simulink model "MtrCtrl_24V_2018"  (R2018b)
settings: Solver=FixedStepDiscrete  StartTime=0.0  StopTime=1  FixedStep=1e-6  RelTol=1e-3
values from neighbouring files (symbols this model uses):
  B = 0.001889    [MtrCtrl_v01.sldd]
  C_LUT_AngleTable_sng_Null = 0.0015339807878856412 0.0030679615757712823 0.0046019423636569235 0.0061359231515425647 0.0076699039394282058 0.009203884727313847 0.010737865515199488 0.012271846303085129 0.013805827090970771 0.015339807878856412 0.016873788666742051 0.018407769454627694 0.019941750242513337 0.021475731030398976 0.023009711818284616 0.024543692606170259 0.0260776733940559 0.027611654181941541 0.02914563496982718    [MtrCtrl_v01.sldd]
  C_LUT_SinTable_sng_Null = 0.0015339801862847655 0.0030679567629659761 0.0046019261204485705 0.0061358846491544753 0.007669828739531097 0.00920375478205982 0.010737659167264491 0.012271538285719925 0.013805388528060391 0.0153392062849881 0.01687298794728171 0.01840672990580482 0.019940428551514441 0.021474080275469508 0.023007681468839369 0.024541228522912288 0.0260747178291039 0.02760814577896574 0.029141508764193722 0.030    [MtrCtrl_v01.sldd]
  C_MATH_OneOverSqrtThree_s32n31_Null = 0.57735026918962584    [MtrCtrl_v01.sldd]
  C_MATH_Pi_u32n30_Null = 3.1415926535897931    [MtrCtrl_v01.sldd]
  C_MATH_SqrtThreeOverThree_s32n31_Null = 0.57735026918962573    [MtrCtrl_v01.sldd]
  C_PMSM_CurQKi_u32n31_null = 0.15707963267949    [MtrCtrl_v01.sldd]
  C_PMSM_CurQKp_u32n31_null = 19.949113350295185    [MtrCtrl_v01.sldd]
  C_PMSM_Flux_u32n32_Vs = 0.192    [MtrCtrl_v01.sldd]
  C_PMSM_Ls_pu = 0.398982267005904    [MtrCtrl_v01.sldd]
  C_PMSM_PolePairs_u8_Null = 4.0    [MtrCtrl_v01.sldd]
  Flux = 0.192    [MtrCtrl_v01.sldd]
  IBase_A = 2000.0    [MtrCtrl_v01.sldd]
  J = 0.011    [MtrCtrl_v01.sldd]
  K_CCM_MRASEna_bool_Flg = 0.0    [MtrCtrl_v01.sldd]
  K_SVM_DefultDuty_s32n31_Null = 0.25    [MtrCtrl_v01.sldd]
  KCCM_VirPosn_flg = 0.0    [MtrCtrl_v01.sldd]
  KCCM_VoltModeEna_Flg = 0.0    [MtrCtrl_v01.sldd]
  Kis = 114583.3333333333    [MtrCtrl_v01.sldd]
  KSMO_EnaEst_Flg = 0.0    [MtrCtrl_v01.sldd]
  Kt = 1.1520000000000001    [MtrCtrl_v01.sldd]
  Ld = 0.000635    [MtrCtrl_v01.sldd]
  LPF_coefg = 0.01    [MtrCtrl_v01.sldd]
  Lq = 0.000685    [MtrCtrl_v01.sldd]
  Ls = 0.000635    [MtrCtrl_v01.sldd]
  OneOverUBase_V = 0.0016666666666666668    [MtrCtrl_v01.sldd]
  Pp = 4.0    [MtrCtrl_v01.sldd]
  Rs = 0.05    [MtrCtrl_v01.sldd]
  SecPerRnd = 0.6    [MtrCtrl_v01.sldd]
  SMOGain_V = 323.31615074619043    [MtrCtrl_v01.sldd]
  Ts = 1.0E-6    [MtrCtrl_v01.sldd]
  TsCtrl = 1.0E-6    [MtrCtrl_v01.sldd]
  UBase_V = 600.0    [MtrCtrl_v01.sldd]
  wmBase_rps = 314.15926535897933    [MtrCtrl_v01.sldd]
undefined symbols (not defined in the file or in its folder): DiscIntNeverNeededParam, Ion, Lithium, sinTable
libraries: powerlib x39, simulink x17, ee_lib x16, nesl_utility x6, simulink_extras x2, eePmsmFwController x1, electricdrivelib x1, fl_lib x1
(part 4 of 5)

== system MtrCtrl_24V_2018/CurLpCtrl/Subsystem10/Subsystem ==
  idqRef : Inport  OutDataTypeStr=fixdt(1,32,31)
  vdq : Inport  Port=2  OutDataTypeStr=fixdt(1,32,31)
  VphMax : Inport  Port=3  OutDataTypeStr=fixdt(0,32,32)
  Cartesian to Polar : Subsystem  Tag=DecoupledSystem
  Constant : Constant  Value=C_MATH_Pi_u32n30_Null  OutDataTypeStr=fixdt(0,32,30)  SampleTime=-1
  Demux : Demux  Outputs=2
  Discrete-Time Integrator : DiscreteIntegrator  IntegratorMethod=Integration: Backward Euler  gainval=5  InitialCondition=1  SampleTime=-1  OutDataTypeStr=fixdt(1,32,28)  ICPrevOutput=DiscIntNeverNeededParam  ICPrevScaledInput=DiscIntNeverNeededParam
  Gain : Gain  Gain=50  OutDataTypeStr=fixdt(1,32,25)
  Gain1 : Gain  Gain=10  OutDataTypeStr=fixdt(1,32,25)
  Gain2 : Gain  Gain=2
  Modulation index threshold : Constant  Value=C_MATH_SqrtThreeOverThree_s32n31_Null  OutDataTypeStr=fixdt(0,32,31)  SampleTime=-1
  Modulation index threshold1 : Constant  Value=3.24  OutDataTypeStr=fixdt(0,32,30)  SampleTime=-1
  Mux : Mux  Inputs=2
  Polar to Cartesian : Subsystem  Tag=DecoupledSystem
  Product : Product  OutDataTypeStr=fixdt(1,32,28)
  Saturation : Saturate  UpperLimit=1  LowerLimit=0  OutDataTypeStr=fixdt(1,32,28)
  Subsystem1 : Subsystem
  Sum : Sum  Inputs=|-+  OutDataTypeStr=fixdt(1,32,30)
  Sum1 : Sum  Inputs=|-+  OutDataTypeStr=fixdt(1,32,28)
  Sum2 : Sum  Inputs=|-+  OutDataTypeStr=fixdt(1,32,28)
  Sum3 : Sum  Inputs=-+  OutDataTypeStr=fixdt(1,32,28)
  Sum4 : Sum  Inputs=|++  OutDataTypeStr=fixdt(1,32,25)
  Unit Delay : UnitDelay  SampleTime=-1  HasFrameUpgradeWarning=on
  idqRefFW : Outport  VectorParamsAs1DForOutWhenUnconnected=off
  wires:
  Product/1 -> Sum2/1
  Sum1/1 -> Product/1
  Gain1/1 -> Sum4/2
  Cartesian to Polar/1(Out1) -> Polar to Cartesian/1(In1)
  Subsystem1/1(M) -> Sum/1
  Sum/1 -> Gain/1
  Discrete-Time Integrator/1 -> Saturation/1, Sum3/1
  Unit Delay/1 -> Gain1/1
  Cartesian to Polar/2(Out2) -> Sum1/1
  Polar to Cartesian/2(Out2) -> Mux/2
  Mux/1 -> idqRefFW/1
  Gain/1 -> Sum4/1
  VphMax/1 -> Subsystem1/2(VphMax)
  Modulation index threshold/1 -> Gain2/1
  Saturation/1 -> Product/2, Sum3/2
  Demux/2 -> Cartesian to Polar/2(In2)
  Demux/1 -> Cartesian to Polar/1(In1)
  idqRef/1 -> Demux/1
  Polar to Cartesian/1(Out1) -> Mux/1
  Constant/1 -> Sum1/2, Sum2/2
  Sum3/1 -> Unit Delay/1
  vdq/1 -> Subsystem1/1(vdq)
  Sum2/1 -> Polar to Cartesian/2(In2)
  Sum4/1 -> Discrete-Time Integrator/1
  Gain2/1 -> Sum/2

== system MtrCtrl_24V_2018/CurLpCtrl/Subsystem2/Subsystem1 ==
  In1 : Inport  OutDataTypeStr=fixdt(0,32,0)
  Constant7 : Constant  Value=2*pi  OutDataTypeStr=fixdt(0,32,0)
  Mod : Math  Operator=mod  SaturateOnIntegerOverflow=on
  Out1 : Outport
  wires:
  Mod/1 -> Out1/1
  In1/1 -> Mod/1
  Constant7/1 -> Mod/2

== system MtrCtrl_24V_2018/CurLpCtrl/Subsystem2/Subsystem2 ==
  FilterIn : Inport  OutDataTypeStr=fixdt(1,32,31)
  Rest : Inport  Port=2  OutDataTypeStr=fixdt(1,32,0)
  Add : Sum  Inputs=+-  OutDataTypeStr=fixdt(1,32,31)
  Add1 : Sum  OutDataTypeStr=fixdt(1,32,31)
  Constant : Constant  Value=LPF_coefg  OutDataTypeStr=fixdt(0,32,31)
  Delay : Delay  DelayLength=1  ExternalReset=Either
      settings: InputPortMap=u0,r5
  Product : Product  OutDataTypeStr=fixdt(1,32,31)
  FilterOut : Outport
  wires:
  FilterIn/1 -> Add/1
  Add/1 -> Product/2
  Product/1 -> Add1/1
  Add1/1 -> Delay/1, FilterOut/1
  Delay/1 -> Add/2, Add1/2
  Rest/1 -> Delay/2
  Constant/1 -> Product/1

== system MtrCtrl_24V_2018/CurLpCtrl/Subsystem2/Subsystem3 ==
  ParkPosn : Inport  OutDataTypeStr=fixdt(1,32,28)
  1-D Lookup Table : Lookup_n-D  NumberOfTableDimensions=1  BreakpointsForDimension1=sinTable(2,:)  BeginIndexSearchUsingPreviousIndexResult=on  Table=sinTable(1,:)  ExtrapMethod=Clip  UseLastTableValue=on  InternalRulePriority=Speed  OutDataTypeStr=fixdt(0,32,31)  RndMeth=Simplest  InputSameDT=on
  1-D Lookup Table1 : Lookup_n-D  NumberOfTableDimensions=1  BreakpointsForDimension1=sinTable(2,:)  BeginIndexSearchUsingPreviousIndexResult=on  Table=sinTable(1,:)  ExtrapMethod=Clip  UseLastTableValue=on  InternalRulePriority=Speed  OutDataTypeStr=fixdt(0,32,31)  RndMeth=Simplest  InputSameDT=on
  Add : Sum  OutDataTypeStr=fixdt(1,32,26)
  Chart : Stateflow chart  TreatAsAtomicUnit=on
  Constant1 : Constant  Value=0  OutDataTypeStr=fixdt(1,32,4)
  Gain : Gain  Gain=4  OutDataTypeStr=fixdt(1,32,26)
  Product : Product  OutDataTypeStr=fixdt(1,32,30)  RndMeth=Simplest
  Product1 : Product  OutDataTypeStr=fixdt(1,32,30)
  Scope : Scope  NumInputPorts=3
  SinTheta : Outport
  CosTheta : Outport  Port=2
  wires:
  ParkPosn/1 -> Gain/1
  Gain/1 -> Add/2
  Constant1/1 -> Add/1
  Product/1 -> Scope/1, SinTheta/1
  Product1/1 -> Scope/2, CosTheta/1
  Add/1 -> Scope/3, Chart/1(Angle)
  Chart/1(SinAngle) -> 1-D Lookup Table/1
  Chart/3(CosAngle) -> 1-D Lookup Table1/1
  1-D Lookup Table/1 -> Product/1
  Chart/2(SinSign) -> Product/2
  1-D Lookup Table1/1 -> Product1/1
  Chart/4(CosSign) -> Product1/2

== system MtrCtrl_24V_2018/CurLpCtrl/Subsystem2/Subsystem4 ==
  FilterIn : Inport  OutDataTypeStr=fixdt(1,32,31)
  Rest : Inport  Port=2  OutDataTypeStr=fixdt(1,32,0)
  Add : Sum  Inputs=+-  OutDataTypeStr=fixdt(1,32,31)
  Add1 : Sum  OutDataTypeStr=fixdt(1,32,31)
  Constant : Constant  Value=LPF_coefg  OutDataTypeStr=fixdt(0,32,31)
  Delay : Delay  DelayLength=1  ExternalReset=Either
      settings: InputPortMap=u0,r5
  Product : Product  OutDataTypeStr=fixdt(1,32,31)
  FilterOut : Outport
  wires:
  Rest/1 -> Delay/2
  Delay/1 -> Add1/2, Add/2
  Add1/1 -> FilterOut/1, Delay/1
  Product/1 -> Add1/1
  Add/1 -> Product/2
  FilterIn/1 -> Add/1
  Constant/1 -> Product/1

== system MtrCtrl_24V_2018/CurLpCtrl/Subsystem2/Subsystem5 ==
  FilterIn : Inport  OutDataTypeStr=fixdt(1,32,22)
  Rest : Inport  Port=2  OutDataTypeStr=fixdt(1,32,0)
  Add : Sum  Inputs=+-  OutDataTypeStr=fixdt(1,32,23)
  Add1 : Sum  OutDataTypeStr=fixdt(1,32,22)
  Constant : Constant  Value=LPF_coefg  OutDataTypeStr=fixdt(0,32,38)
  Delay : Delay  DelayLength=1  ExternalReset=Either
      settings: InputPortMap=u0,r5
  Product : Product  OutDataTypeStr=fixdt(1,32,29)
  FilterOut : Outport
  wires:
  FilterIn/1 -> Add/1
  Add/1 -> Product/2
  Product/1 -> Add1/1
  Add1/1 -> Delay/1, FilterOut/1
  Delay/1 -> Add/2, Add1/2
  Rest/1 -> Delay/2
  Constant/1 -> Product/1

== system MtrCtrl_24V_2018/CurLpCtrl/Subsystem2/Z_alpha ==
  Salpha : Inport  OutDataTypeStr=int32
  Constant : Constant  OutDataTypeStr=fixdt(1,32,30)
  Constant1 : Constant  Value=-1  OutDataTypeStr=fixdt(1,32,30)
  Divide : Product  Inputs=*/  OutDataTypeStr=fixdt(1,32,30)
  E : Constant  Value=600  OutDataTypeStr=int32
  If : If  NumInputs=2  IfExpression=u1 > u2  ElseIfExpressions=u1 < -u2
  If Action Subsystem : Subsystem  TreatAsAtomicUnit=on
  If Action Subsystem1 : Subsystem  TreatAsAtomicUnit=on
  If Action Subsystem2 : Subsystem  TreatAsAtomicUnit=on
  Merge : Merge  Inputs=3
  ZalphaOut : Outport
  wires:
  Salpha/1 -> If/1, Divide/1
  E/1 -> If/2, Divide/2
  Divide/1 -> If Action Subsystem2/1(In1)
  If/1 -> If Action Subsystem/Action
  If Action Subsystem/1(ZalphaOut) -> Merge/1
  If/3 -> If Action Subsystem2/Action
  If/2 -> If Action Subsystem1/Action
  If Action Subsystem1/1(ZalphaOut) -> Merge/2
  If Action Subsystem2/1(ZalphaOut) -> Merge/3
  Merge/1 -> ZalphaOut/1
  Constant/1 -> If Action Subsystem/1(In1)
  Constant1/1 -> If Action Subsystem1/1(In1)

== system MtrCtrl_24V_2018/CurLpCtrl/Subsystem2/Z_alpha1 ==
  Salpha : Inport  OutDataTypeStr=int32
  Constant : Constant  OutDataTypeStr=fixdt(1,32,30)
  Constant1 : Constant  Value=-1  OutDataTypeStr=fixdt(1,32,30)
  Divide : Product  Inputs=*/  OutDataTypeStr=fixdt(1,32,30)
  E : Constant  Value=600  OutDataTypeStr=int32
  If : If  NumInputs=2  IfExpression=u1 > u2  ElseIfExpressions=u1 < -u2
  If Action Subsystem : Subsystem  TreatAsAtomicUnit=on
  If Action Subsystem1 : Subsystem  TreatAsAtomicUnit=on
  If Action Subsystem2 : Subsystem  TreatAsAtomicUnit=on
  Merge : Merge  Inputs=3
  ZalphaOut : Outport
  wires:
  Constant1/1 -> If Action Subsystem1/1(In1)
  Constant/1 -> If Action Subsystem/1(In1)
  Merge/1 -> ZalphaOut/1
  If Action Subsystem2/1(ZalphaOut) -> Merge/3
  If Action Subsystem1/1(ZalphaOut) -> Merge/2
  If/2 -> If Action Subsystem1/Action
  If/3 -> If Action Subsystem2/Action
  If Action Subsystem/1(ZalphaOut) -> Merge/1
  If/1 -> If Action Subsystem/Action
  Divide/1 -> If Action Subsystem2/1(In1)
  E/1 -> Divide/2, If/2
  Salpha/1 -> Divide/1, If/1

== system MtrCtrl_24V_2018/CurLpCtrl/Subsystem4/SinCos ==
  In1 : Inport  LockScale=on
  DTC_input_1 : DataTypeConversion  OutDataTypeStr=fixdt('double')  RndMeth=Nearest  LockScale=on
  DTC_output_1 : DataTypeConversion  OutDataTypeStr=fixdt(1,32,4)
  DTC_output_2 : DataTypeConversion  OutDataTypeStr=fixdt(0,32,31)
  ReplicaOfSource : Trigonometry  Operator=sincos
  Out1 : Outport  LockScale=on
  Out2 : Outport  Port=2  LockScale=on
  wires:
  In1/1 -> DTC_input_1/1
  DTC_output_1/1 -> Out1/1
  ReplicaOfSource/1 -> DTC_output_1/1
  ReplicaOfSource/2 -> DTC_output_2/1
  DTC_input_1/1 -> ReplicaOfSource/1
  DTC_output_2/1 -> Out2/1

== system MtrCtrl_24V_2018/CurLpCtrl/Subsystem8/F12 ==
  we : Inport
  Dlt_Ud_k : Inport  Port=2
  Dlt_Uq_k : Inport  Port=3
  Add{2..5} (4 alike) : Sum
  Constant1 : Constant  Value=-TsCtrl*Rs/Ls
  Constant14 : Constant  Value=-TsCtrl*Rs/Ls
  Constant16 : Constant  Value=TsCtrl/Ls
  Constant2 : Constant  Value=TsCtrl/Ls
  Discrete-Time Integrator : DiscreteIntegrator  SampleTime=-1  ICPrevOutput=DiscIntNeverNeededParam  ICPrevScaledInput=DiscIntNeverNeededParam
  Discrete-Time Integrator1 : DiscreteIntegrator  SampleTime=-1  ICPrevOutput=DiscIntNeverNeededParam  ICPrevScaledInput=DiscIntNeverNeededParam
  Gain6 : Gain  Gain=TsCtrl
  Gain7 : Gain  Gain=-1
  Product{5,9..13} (6 alike) : Product
  Dlt_Id : Outport
  Dlt_Iq : Outport  Port=2
  wires:
  Dlt_Ud_k/1 -> Product12/2
  Product13/1 -> Add5/2
  Add4/1 -> Discrete-Time Integrator/1  "Id_k2"
  Add3/1 -> Add5/1
  Constant14/1 -> Product5/2
  Gain7/1 -> Product10/1
  we/1 -> Gain6/1
  Add5/1 -> Discrete-Time Integrator1/1  "Iq_k2"
  [Dlt_Iq] -> Product9/1, Product11/2
  Add2/1 -> Add4/1
  Constant16/1 -> Product12/1
  Product11/1 -> Add3/2
  [Dlt_Id] -> Product5/1, Product10/2
  Product12/1 -> Add4/2
  Product9/1 -> Add2/2
  Product5/1 -> Add2/1
  Dlt_Uq_k/1 -> Product13/2
  Constant1/1 -> Product11/1
  Gain6/1 -> Product9/2, Gain7/1
  Product10/1 -> Add3/1
  Constant2/1 -> Product13/1
  Discrete-Time Integrator/1 -> [Dlt_Id], Dlt_Id/1
  Discrete-Time Integrator1/1 -> [Dlt_Iq], Dlt_Iq/1

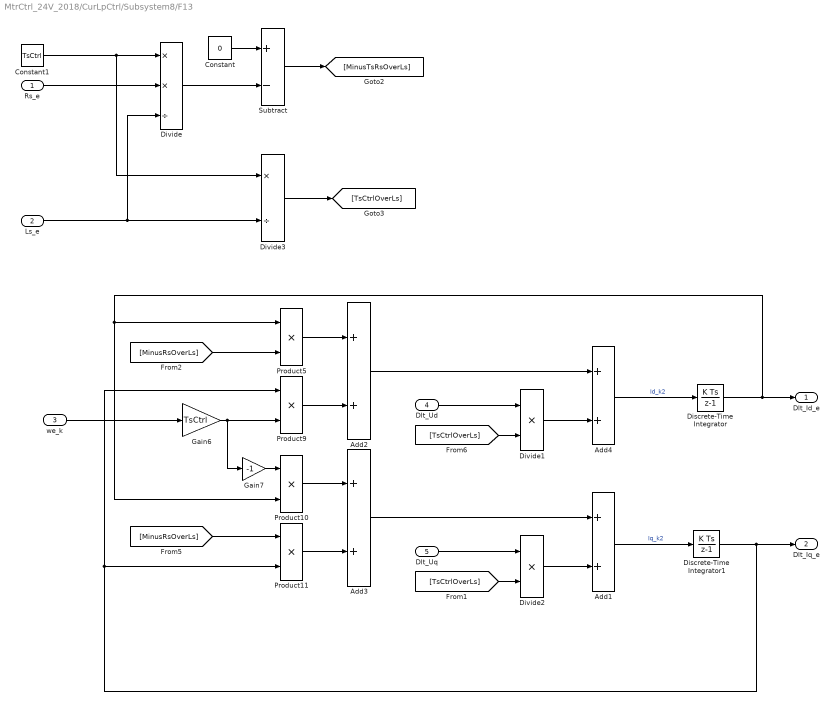
== system MtrCtrl_24V_2018/CurLpCtrl/Subsystem8/F13 ==
  Rs_e : Inport
  Ls_e : Inport  Port=2
  we_k : Inport  Port=3
  Dlt_Ud : Inport  Port=4
  Dlt_Uq : Inport  Port=5
  Add{1..4} (4 alike) : Sum
  Constant : Constant  Value=0
  Constant1 : Constant  Value=TsCtrl
  Discrete-Time Integrator : DiscreteIntegrator  SampleTime=-1  ICPrevOutput=DiscIntNeverNeededParam  ICPrevScaledInput=DiscIntNeverNeededParam
  Discrete-Time Integrator1 : DiscreteIntegrator  SampleTime=-1  ICPrevOutput=DiscIntNeverNeededParam  ICPrevScaledInput=DiscIntNeverNeededParam
  Divide : Product  Inputs=**/
  Divide1 : Product  Inputs=**
  Divide2 : Product  Inputs=**
  Divide3 : Product  Inputs=*/
  Gain6 : Gain  Gain=TsCtrl
  Gain7 : Gain  Gain=-1
  Product{5,9..11} (4 alike) : Product
  Subtract : Sum  Inputs=+-
  Dlt_Id_e : Outport
  Dlt_Iq_e : Outport  Port=2
  wires:
  Dlt_Ud/1 -> Divide1/1
  Divide2/1 -> Add1/2
  Add4/1 -> Discrete-Time Integrator/1  "Id_k2"
  Add3/1 -> Add1/1
  [MinusRsOverLs] -> Product5/2
  Gain7/1 -> Product10/1
  we_k/1 -> Gain6/1
  Add1/1 -> Discrete-Time Integrator1/1  "Iq_k2"
  Discrete-Time Integrator1/1 -> Dlt_Iq_e/1, Product9/1, Product11/2
  Add2/1 -> Add4/1
  [TsCtrlOverLs] -> Divide1/2
  Product11/1 -> Add3/2
  Discrete-Time Integrator/1 -> Product5/1, Product10/2, Dlt_Id_e/1
  Divide1/1 -> Add4/2
  Product9/1 -> Add2/2
  Product5/1 -> Add2/1
  Dlt_Uq/1 -> Divide2/1
  [MinusRsOverLs] -> Product11/1
  Gain6/1 -> Product9/2, Gain7/1
  Product10/1 -> Add3/1
  Constant/1 -> Subtract/1
  Rs_e/1 -> Divide/2
  Divide/1 -> Subtract/2
  Subtract/1 -> [MinusTsRsOverLs]
  Ls_e/1 -> Divide3/2, Divide/3
  [TsCtrlOverLs] -> Divide2/2
  Constant1/1 -> Divide3/1, Divide/1
  Divide3/1 -> [TsCtrlOverLs]

== system MtrCtrl_24V_2018/CurLpCtrl/Subsystem8/F15 ==
  Id : Inport
  Iq : Inport  Port=2
  Id_e : Inport  Port=3
  Iq_e : Inport  Port=4
  Add : Sum
  Constant2 : Constant  Value=10
  Constant3 : Constant  Value=0
  Constant8 : Constant  Commented=on  Value=2*Rs/Ls
  Gain : Gain  Gain=-1
  PID Controller : simulink/Continuous/PID Controller  Controller=PI  Form=Parallel  TimeDomain=Discrete-time  SampleTime=-1  IntegratorMethod=Forward Euler  ControllerParametersSource=external  P=1  I=1  D=0  N=100  UseFilter=on  TunerSelectOption=Transfer Function Based (PID Tuner App)  InitialConditionSource=internal  InitialConditionForIntegrator=0  InitialConditionForFilter=0  DifferentiatorICPrevScaledInput=0  ExternalReset=none  TrackingMode=off  Kt=1  LimitOutput=off  UpperSaturationLimit=inf  LowerSaturationLimit=-inf  LinearizeAsGain=on  AntiWindupMode=none  Kb=1  POutMin=[]  POutMax=[]  IOutMin=[]  IOutMax=[]  DOutMin=[]  DOutMax=[]  NOutMin=[]  NOutMax=[]  SumOutMin=[]  SumOutMax=[]  SaturationOutMin=[]  SaturationOutMax=[]  PParamMin=[]  PParamMax=[]  IParamMin=[]  IParamMax=[]  DParamMin=[]  DParamMax=[]  NParamMin=[]  NParamMax=[]  KbParamMin=[]  KbParamMax=[]  KtParamMin=[]  KtParamMax=[]  KbOutMin=[]  KbOutMax=[]  KtOutMin=[]  KtOutMax=[]  IntegratorOutMin=[]  IntegratorOutMax=[]  FilterOutMin=[]  FilterOutMax=[]  SumI1OutMin=[]  SumI1OutMax=[]  SumI2OutMin=[]  SumI2OutMax=[]  SumI3OutMin=[]  SumI3OutMax=[]  SumI4OutMin=[]  SumI4OutMax=[]  SumDOutMin=[]  SumDOutMax=[]  DifferentiatorOutMin=[]  DifferentiatorOutMax=[]  FilterDiffOutCoefMin=[]  FilterDiffOutCoefMax=[]  ReciprocalOutMin=[]  ReciprocalOutMax=[]  SumDenOutMin=[]  SumDenOutMax=[]  SumNumOutMin=[]  SumNumOutMax=[]  DivideOutMin=[]  DivideOutMax=[]  IntegratorContinuousStateAttributes=''  IntegratorStateMustResolveToSignalObject=off  IntegratorRTWStateStorageClass=Auto  FilterContinuousStateAttributes=''  FilterStateMustResolveToSignalObject=off  FilterRTWStateStorageClass=Auto  ParallelPVariant=ExternalParameters  IdealPVariant=Disabled  IVariant=ExternalParameters  DVariant=Disabled  IntegratorVariant=Discrete  SatVariant=Disabled  AWVariant=Passthrough  PCopyVariant=Disabled  TRVariant=Disabled  FdbkBlocksVariant=Forward  IdealPFdbkVariant=Disabled  SatFdbkVariant=Disabled  DerivativeFilterVariant=Disabled  NVariant=Disabled  NCopyVariant=Disabled_SignalSpec  FilterICVariant=Disabled  IntegratorICVariant=InternalICs  ExternalResetVariant=Disabled  TRSumVariant=Passthrough  SumFdbkVariant=Disabled  SumVariant=Sum_PI
  Product3 : Product
  Product5 : Product
  Subtract6 : Sum  Inputs=+-
  Subtract7 : Sum  Inputs=+-
  Rs/Ls : Outport
  wires:
  Iq/1 -> Subtract7/1
  Id/1 -> Subtract6/1
  Constant8/1 -> ?
  Product3/1 -> Add/1
  Subtract6/1 -> Product3/1
  Product5/1 -> Add/2
  Iq_e/1 -> Subtract7/2, Product5/2
  Subtract7/1 -> Product5/1
  Id_e/1 -> Product3/2, Subtract6/2
  PID Controller/1 -> Gain/1
  Constant2/1 -> PID Controller/2
  Add/1 -> PID Controller/1
  Constant3/1 -> PID Controller/3
  Gain/1 -> Rs/Ls/1

== system MtrCtrl_24V_2018/CurLpCtrl/Subsystem8/F16 ==
  Id : Inport
  Iq : Inport  Port=2
  Id_e : Inport  Port=3
  Iq_e : Inport  Port=4
  Ud : Inport  Port=5
  Uq : Inport  Port=6
  Add : Sum
  Constant2 : Constant  Value=10
  Constant3 : Constant  Value=0
  PID Controller : simulink/Continuous/PID Controller  Controller=PI  Form=Parallel  TimeDomain=Discrete-time  SampleTime=-1  IntegratorMethod=Forward Euler  ControllerParametersSource=external  P=1  I=1  D=0  N=100  UseFilter=on  TunerSelectOption=Transfer Function Based (PID Tuner App)  InitialConditionSource=internal  InitialConditionForIntegrator=0  InitialConditionForFilter=0  DifferentiatorICPrevScaledInput=0  ExternalReset=none  TrackingMode=off  Kt=1  LimitOutput=off  UpperSaturationLimit=inf  LowerSaturationLimit=-inf  LinearizeAsGain=on  AntiWindupMode=none  Kb=1  POutMin=[]  POutMax=[]  IOutMin=[]  IOutMax=[]  DOutMin=[]  DOutMax=[]  NOutMin=[]  NOutMax=[]  SumOutMin=[]  SumOutMax=[]  SaturationOutMin=[]  SaturationOutMax=[]  PParamMin=[]  PParamMax=[]  IParamMin=[]  IParamMax=[]  DParamMin=[]  DParamMax=[]  NParamMin=[]  NParamMax=[]  KbParamMin=[]  KbParamMax=[]  KtParamMin=[]  KtParamMax=[]  KbOutMin=[]  KbOutMax=[]  KtOutMin=[]  KtOutMax=[]  IntegratorOutMin=[]  IntegratorOutMax=[]  FilterOutMin=[]  FilterOutMax=[]  SumI1OutMin=[]  SumI1OutMax=[]  SumI2OutMin=[]  SumI2OutMax=[]  SumI3OutMin=[]  SumI3OutMax=[]  SumI4OutMin=[]  SumI4OutMax=[]  SumDOutMin=[]  SumDOutMax=[]  DifferentiatorOutMin=[]  DifferentiatorOutMax=[]  FilterDiffOutCoefMin=[]  FilterDiffOutCoefMax=[]  ReciprocalOutMin=[]  ReciprocalOutMax=[]  SumDenOutMin=[]  SumDenOutMax=[]  SumNumOutMin=[]  SumNumOutMax=[]  DivideOutMin=[]  DivideOutMax=[]  IntegratorContinuousStateAttributes=''  IntegratorStateMustResolveToSignalObject=off  IntegratorRTWStateStorageClass=Auto  FilterContinuousStateAttributes=''  FilterStateMustResolveToSignalObject=off  FilterRTWStateStorageClass=Auto  ParallelPVariant=ExternalParameters  IdealPVariant=Disabled  IVariant=ExternalParameters  DVariant=Disabled  IntegratorVariant=Discrete  SatVariant=Disabled  AWVariant=Passthrough  PCopyVariant=Disabled  TRVariant=Disabled  FdbkBlocksVariant=Forward  IdealPFdbkVariant=Disabled  SatFdbkVariant=Disabled  DerivativeFilterVariant=Disabled  NVariant=Disabled  NCopyVariant=Disabled_SignalSpec  FilterICVariant=Disabled  IntegratorICVariant=InternalICs  ExternalResetVariant=Disabled  TRSumVariant=Passthrough  SumFdbkVariant=Disabled  SumVariant=Sum_PI
  Product3 : Product
  Product5 : Product
  Scope : Scope
  Subtract6 : Sum  Inputs=+-
  Subtract7 : Sum  Inputs=+-
  1/Ls : Outport
  wires:
  Id_e/1 -> Subtract6/2
  Subtract7/1 -> Product5/1
  Iq_e/1 -> Subtract7/2
  Product5/1 -> Add/2
  Subtract6/1 -> Product3/1
  Product3/1 -> Add/1
  Id/1 -> Subtract6/1
  Iq/1 -> Subtract7/1
  Ud/1 -> Product3/2
  Uq/1 -> Product5/2
  PID Controller/1 -> 1/Ls/1, Scope/1
  Constant3/1 -> PID Controller/3
  Add/1 -> PID Controller/1
  Constant2/1 -> PID Controller/2

== system MtrCtrl_24V_2018/CurLpCtrl/Subsystem8/F9 ==
  Id_k : Inport
  Iq_k : Inport  Port=2
  we : Inport  Port=3
  Ud_k : Inport  Port=4
  Uq_k : Inport  Port=5
  Delay{1..4} (4 alike) : Delay  DelayLength=1
  F2 : Subsystem
  F8 : Subsystem
  Subtract : Sum  Inputs=+-
  Subtract1 : Sum  Inputs=+-
  Id_k_1 : Outport
  Iq_k_1 : Outport  Port=2
  Dlt_Id_k_1 : Outport  Port=3
  Id_k_e : Outport  Port=4
  Iq_k_e : Outport  Port=5
  Dlt_Iq_k_1 : Outport  Port=6
  wires:
  Id_k/1 -> Delay1/1, F2/1(Id_k)
  Iq_k/1 -> Delay4/1, F2/2(Iq_k)
  Subtract/1 -> Dlt_Id_k_1/1
  Subtract1/1 -> Dlt_Iq_k_1/1
  we/1 -> F2/3(we), F8/3(we)
  Ud_k/1 -> Delay2/1, F2/4(Ud_k)
  Uq_k/1 -> Delay3/1, F2/5(Uq_k)
  Delay2/1 -> F8/4(Ud_k1)
  Delay3/1 -> F8/5(Uq_k1)
  F8/1(Id_k) -> Subtract/2, Id_k_e/1
  F8/2(Iq_k) -> Iq_k_e/1, Subtract1/2
  F2/1(Id_k_1) -> Id_k_1/1, Subtract/1
  F2/2(Iq_k_1) -> Iq_k_1/1, Subtract1/1
  Delay1/1 -> F8/1(Id_k1)
  Delay4/1 -> F8/2(Iq_k1)

== system MtrCtrl_24V_2018/Inverter/Subsystem/Subsystem1 ==
  CaptureEna : Inport
  Add : Sum
  Constant : Constant  Value=2.5
  Constant1 : Constant  Value=5
  Constant2 : Constant  Value=4096
  Constant3 : Constant  Value=2048
  Constant4 : Constant  Value=0.2442
  Divide : Product  Inputs=*/  OutDataTypeStr=single
  Product : Product  OutDataTypeStr=single
  Product1 : Product  OutDataTypeStr=single
  Subtract : Sum  Inputs=+-  OutDataTypeStr=single
  Switch : Switch  Criteria=u2 > Threshold
  Voltage Measurement : powerlib/Measurements/Voltage Measurement  PhasorSimulation=off  OutputType=Complex  PSBequivalent=0
  - : PMIOPort  Side=Left
  + : PMIOPort  Port=2  Side=Left
  CurC_Cap : Outport
  wires:
  Add/1 -> Switch/1
  Constant3/1 -> Subtract/2
  Product/1 -> Subtract/1
  Divide/1 -> Product/2
  Constant/1 -> Add/2, Switch/3
  Subtract/1 -> Product1/1  "CurC_ADC"
  Voltage Measurement/1 -> Add/1
  Constant1/1 -> Divide/2
  Constant4/1 -> Product1/2
  Switch/1 -> Divide/1
  Constant2/1 -> Product/1
  Product1/1 -> CurC_Cap/1  "CurC_LowTerCap"
  CaptureEna/1 -> Switch/2
  connections:
  Voltage Measurement/LConn2 -- -/RConn1
  Voltage Measurement/LConn1 -- +/RConn1

== system MtrCtrl_24V_2018/Inverter/Subsystem/Subsystem4 ==
  CaptureEna : Inport
  Add : Sum
  Constant : Constant  Value=2.5
  Constant1 : Constant  Value=5
  Constant2 : Constant  Value=4096
  Constant3 : Constant  Value=2048
  Constant4 : Constant  Value=1.221
  Divide : Product  Inputs=*/
  Product : Product
  Product1 : Product  OutDataTypeStr=single
  Subtract : Sum  Inputs=+-  OutDataTypeStr=single
  Switch : Switch  Criteria=u2 > Threshold
  Voltage Measurement : powerlib/Measurements/Voltage Measurement  PhasorSimulation=off  OutputType=Complex  PSBequivalent=0
  - : PMIOPort  Side=Left
  + : PMIOPort  Port=2  Side=Left
  CurC_Cap : Outport
  wires:
  CaptureEna/1 -> Switch/2
  Product1/1 -> CurC_Cap/1  "CurC_LowTerCap"
  Constant2/1 -> Product/1
  Switch/1 -> Divide/1
  Constant4/1 -> Product1/2
  Constant1/1 -> Divide/2
  Voltage Measurement/1 -> Add/1
  Subtract/1 -> Product1/1  "CurC_ADC"
  Constant/1 -> Switch/3, Add/2
  Divide/1 -> Product/2
  Product/1 -> Subtract/1
  Constant3/1 -> Subtract/2
  Add/1 -> Switch/1
  connections:
  Voltage Measurement/LConn1 -- +/RConn1
  Voltage Measurement/LConn2 -- -/RConn1

== system MtrCtrl_24V_2018/Inverter/Subsystem/Subsystem5 ==
  CaptureEna : Inport
  Add : Sum
  Constant : Constant  Value=2.5
  Constant1 : Constant  Value=5
  Constant2 : Constant  Value=4096
  Constant3 : Constant  Value=2048
  Constant4 : Constant  Value=1.221
  Divide : Product  Inputs=*/
  Product : Product
  Product1 : Product  OutDataTypeStr=single
  Subtract : Sum  Inputs=+-  OutDataTypeStr=single
  Switch : Switch  Criteria=u2 > Threshold
  Voltage Measurement : powerlib/Measurements/Voltage Measurement  PhasorSimulation=off  OutputType=Complex  PSBequivalent=0
  - : PMIOPort  Side=Left
  + : PMIOPort  Port=2  Side=Left
  CurB_Cap : Outport
  wires:
  Add/1 -> Switch/1
  Constant3/1 -> Subtract/2
  Product/1 -> Subtract/1
  Divide/1 -> Product/2
  Constant/1 -> Add/2, Switch/3
  Subtract/1 -> Product1/1  "CurC_ADC"
  Voltage Measurement/1 -> Add/1
  Constant1/1 -> Divide/2
  Constant4/1 -> Product1/2
  Switch/1 -> Divide/1
  Constant2/1 -> Product/1
  Product1/1 -> CurB_Cap/1  "CurB_Cap"
  CaptureEna/1 -> Switch/2
  connections:
  Voltage Measurement/LConn2 -- -/RConn1
  Voltage Measurement/LConn1 -- +/RConn1

== system MtrCtrl_24V_2018/Inverter/Subsystem/Subsystem6 ==
  CaptureEna : Inport
  Add : Sum
  Constant : Constant  Value=2.5
  Constant1 : Constant  Value=5
  Constant2 : Constant  Value=4096
  Constant3 : Constant  Value=2048
  Constant4 : Constant  Value=1.221
  Divide : Product  Inputs=*/
  Product : Product
  Product1 : Product  OutDataTypeStr=single
  Subtract : Sum  Inputs=+-  OutDataTypeStr=single
  Switch : Switch  Criteria=u2 > Threshold
  Voltage Measurement : powerlib/Measurements/Voltage Measurement  PhasorSimulation=off  OutputType=Complex  PSBequivalent=0
  - : PMIOPort  Side=Left
  + : PMIOPort  Port=2  Side=Left
  CurA_Cap : Outport
  wires:
  Add/1 -> Switch/1
  Constant3/1 -> Subtract/2
  Product/1 -> Subtract/1
  Divide/1 -> Product/2
  Constant/1 -> Add/2, Switch/3
  Subtract/1 -> Product1/1  "CurC_ADC"
  Voltage Measurement/1 -> Add/1
  Constant1/1 -> Divide/2
  Constant4/1 -> Product1/2
  Switch/1 -> Divide/1
  Constant2/1 -> Product/1
  Product1/1 -> CurA_Cap/1  "CurA_LowTerCap"
  CaptureEna/1 -> Switch/2
  connections:
  Voltage Measurement/LConn2 -- -/RConn1
  Voltage Measurement/LConn1 -- +/RConn1

== system MtrCtrl_24V_2018/MotorModel/Subsystem/ClarkeTF ==
  Va : Inport
  Vb : Inport  Port=2
  Add : Sum  Inputs=+++
  Gain : Gain  Gain=1/sqrt(3)
  V_alpha : Outport
  V_beta : Outport  Port=2
  wires:
  Add/1 -> Gain/1
  Vb/1 -> Add/3, Add/2
  Va/1 -> V_alpha/1, Add/1
  Gain/1 -> V_beta/1

== system MtrCtrl_24V_2018/MotorModel/Subsystem/InversePark ==
  D : Inport
  Q : Inport  Port=2
  SinTheta : Inport  Port=3
  CosTheta : Inport  Port=4
  Scope : Scope  NumInputPorts=2
  dcos : Product  RndMeth=Simplest  OutDataTypeStr=Inherit: Same as first input
  dsin : Product  RndMeth=Simplest  OutDataTypeStr=Inherit: Same as first input
  qcos : Product  RndMeth=Simplest  OutDataTypeStr=Inherit: Same as first input
  qsin : Product  RndMeth=Simplest  OutDataTypeStr=Inherit: Same as first input
  sum_alpha : Sum  Inputs=|+-  RndMeth=Simplest  OutDataTypeStr=Inherit: Same as first input
  sum_beta : Sum  Inputs=|++  RndMeth=Simplest  OutDataTypeStr=Inherit: Same as first input
  Alpha : Outport
  Beta : Outport  Port=2
  wires:
  sum_alpha/1 -> Scope/1, Alpha/1
  sum_beta/1 -> Scope/2, Beta/1
  dsin/1 -> sum_beta/2
  qcos/1 -> sum_beta/1
  CosTheta/1 -> dcos/2, qcos/2
  qsin/1 -> sum_alpha/2
  SinTheta/1 -> qsin/2, dsin/2
  Q/1 -> qcos/1, qsin/1
  dcos/1 -> sum_alpha/1
  D/1 -> dsin/1, dcos/1

== system MtrCtrl_24V_2018/MotorModel/Subsystem/ParkTF ==
  Valpha : Inport
  Vbeta : Inport  Port=2
  SinTheta : Inport  Port=3
  CosTheta : Inport  Port=4
  Add : Sum
  Add1 : Sum  Inputs=+-
  Product{,1..3} (4 alike) : Product
  Vd : Outport
  Vq : Outport  Port=2
  wires:
  Product/1 -> Add/1
  Product1/1 -> Add/2
  Add/1 -> Vd/1
  Add1/1 -> Vq/1
  Product3/1 -> Add1/1
  Product2/1 -> Add1/2
  Valpha/1 -> Product2/1, Product/1
  SinTheta/1 -> Product2/2, Product1/2
  Vbeta/1 -> Product1/1, Product3/1
  CosTheta/1 -> Product/2, Product3/2

== system MtrCtrl_24V_2018/MotorModel/Subsystem/Subsystem ==
  Vd : Inport
  Vq : Inport  Port=2
  we : Inport  Port=3
  Add : Sum  Inputs=+-+
  Add1 : Sum  Inputs=---+
  Constant : Constant  Value=Lq
  Constant1 : Constant  Value=Rs
  Constant2 : Constant  Value=1/Ld
  Constant3 : Constant  Value=Ld
  Constant4 : Constant  Value=Rs
  Constant5 : Constant  Value=1/Lq
  Constant6 : Constant  Value=Flux
  Discrete-Time Integrator : DiscreteIntegrator  SampleTime=-1  ICPrevOutput=DiscIntNeverNeededParam  ICPrevScaledInput=DiscIntNeverNeededParam
  Discrete-Time Integrator1 : DiscreteIntegrator  SampleTime=-1  ICPrevOutput=DiscIntNeverNeededParam  ICPrevScaledInput=DiscIntNeverNeededParam
  Product : Product  Inputs=3
  Product{1..2,4..6} (5 alike) : Product
  Product3 : Product  Inputs=3
  Scope : Scope
  Id : Outport
  Iq : Outport  Port=2
  wires:
  Discrete-Time Integrator/1 -> Scope/1, Product1/2, Product3/1, Id/1  "Id"
  Vd/1 -> Add/1
  we/1 -> Product6/2, Product3/3, Product/1
  Product5/1 -> Discrete-Time Integrator1/1
  Constant/1 -> Product/2
  Product/1 -> Add/3
  Constant1/1 -> Product1/1
  Product1/1 -> Add/2
  Add/1 -> Product2/1
  Product2/1 -> Discrete-Time Integrator/1
  Constant2/1 -> Product2/2
  Vq/1 -> Add1/4
  Product3/1 -> Add1/2
  Constant3/1 -> Product3/2
  Product4/1 -> Add1/1
  Constant4/1 -> Product4/2
  Constant5/1 -> Product5/2
  Add1/1 -> Product5/1
  Product6/1 -> Add1/3
  Constant6/1 -> Product6/1
  Discrete-Time Integrator1/1 -> Product4/1, Product/3, Iq/1  "Id"

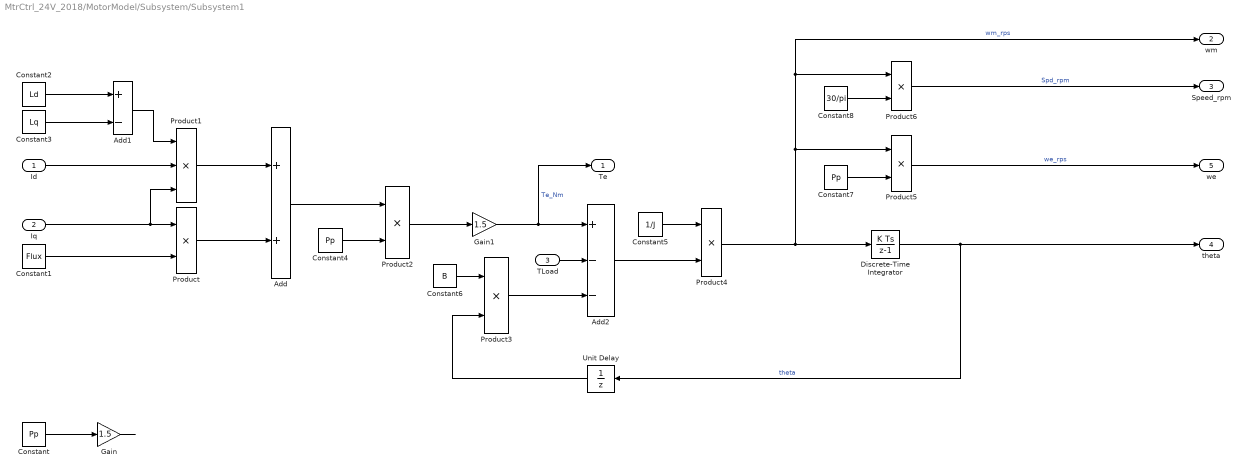
== system MtrCtrl_24V_2018/MotorModel/Subsystem/Subsystem1 ==
  Id : Inport
  Iq : Inport  Port=2
  TLoad : Inport  Port=3
  Add : Sum
  Add1 : Sum  Inputs=+-
  Add2 : Sum  Inputs=+--
  Constant : Constant  Value=Pp
  Constant1 : Constant  Value=Flux
  Constant2 : Constant  Value=Ld
  Constant3 : Constant  Value=Lq
  Constant4 : Constant  Value=Pp
  Constant5 : Constant  Value=1/J
  Constant6 : Constant  Value=B
  Constant7 : Constant  Value=Pp
  Constant8 : Constant  Value=30/pi
  Discrete-Time Integrator : DiscreteIntegrator  SampleTime=-1  ICPrevOutput=DiscIntNeverNeededParam  ICPrevScaledInput=DiscIntNeverNeededParam
  Gain : Gain  Gain=1.5
  Gain1 : Gain  Gain=1.5
  Product{,2..6} (6 alike) : Product
  Product1 : Product  Inputs=3
  Unit Delay : UnitDelay  SampleTime=-1  HasFrameUpgradeWarning=on
  Te : Outport
  wm : Outport  Port=2
  Speed_rpm : Outport  Port=3
  theta : Outport  Port=4
  we : Outport  Port=5
  wires:
  Iq/1 -> Product1/3, Product/1
  Constant/1 -> Gain/1
  Id/1 -> Product1/2
  Constant1/1 -> Product/2
  Gain/1 -> ?
  Product/1 -> Add/2
  Add1/1 -> Product1/1
  Constant2/1 -> Add1/1
  Constant3/1 -> Add1/2
  Product1/1 -> Add/1
  Add/1 -> Product2/1
  Constant4/1 -> Product2/2
  Product2/1 -> Gain1/1
  Gain1/1 -> Add2/1, Te/1  "Te_Nm"
  TLoad/1 -> Add2/2
  Constant7/1 -> Product5/2
  Product5/1 -> we/1  "we_rps"
  Product6/1 -> Speed_rpm/1  "Spd_rpm"
  Constant8/1 -> Product6/2
  Discrete-Time Integrator/1 -> theta/1, Unit Delay/1  "theta"
  Add2/1 -> Product4/2
  Constant5/1 -> Product4/1
  Product4/1 -> Discrete-Time Integrator/1, Product5/1, Product6/1, wm/1  "wm_rps"
  Unit Delay/1 -> Product3/2
  Product3/1 -> Add2/3
  Constant6/1 -> Product3/1

== system MtrCtrl_24V_2018/MotorModel/Subsystem/Subsystem2 ==
  Theta_In : Inport
  Theta_Mtr : Inport  Port=2
  Add : Sum  Inputs=+-
  Constant : Constant  Value=2*pi
  Constant1 : Constant  Value=Pp
  Constant2 : Constant  Value=PosnSelector
  Divide : Product  Inputs=*/  OutDataTypeStr=uint16
  Product : Product
  Product1 : Product
  Scope1 : Scope  NumInputPorts=2
  SinCos : Trigonometry  Operator=sincos
  Switch : Switch  Criteria=u2 > Threshold
  SinTheta : Outport
  CoTheta : Outport  Port=2
  wires:
  Theta_In/1 -> Scope1/1, Switch/1
  Constant/1 -> Product1/2, Divide/2
  Divide/1 -> Product1/1
  Add/1 -> SinCos/1
  Product1/1 -> Add/2
  SinCos/1 -> SinTheta/1
  SinCos/2 -> CoTheta/1
  Theta_Mtr/1 -> Scope1/2, Switch/3
  Constant1/1 -> Product/1
  Product/1 -> Add/1, Divide/1
  Switch/1 -> Product/2
  Constant2/1 -> Switch/2

== system MtrCtrl_24V_2018/MotorModel/Subsystem/Subsystem3 ==
  Alpha : Inport
  Beta : Inport  Port=2
  Add : Sum  Inputs=-+
  Add1 : Sum  Inputs=--
  one_by_two : Gain  Gain=1/2  RndMeth=Simplest  OutDataTypeStr=Inherit: Same as input
  sqrt3_by_two : Gain  Gain=sqrt(3)/2  RndMeth=Simplest  OutDataTypeStr=Inherit: Same as input
  CurA : Outport  VectorParamsAs1DForOutWhenUnconnected=off
  CurB : Outport  Port=2  VectorParamsAs1DForOutWhenUnconnected=off
  CurC : Outport  Port=3  VectorParamsAs1DForOutWhenUnconnected=off
  wires:
  sqrt3_by_two/1 -> Add/2, Add1/2
  Add1/1 -> CurC/1
  one_by_two/1 -> Add/1, Add1/1
  Alpha/1 -> CurA/1, one_by_two/1
  Beta/1 -> sqrt3_by_two/1
  Add/1 -> CurB/1

== system MtrCtrl_24V_2018/CurLpCtrl/SVPWM/Overmodulation/Subsystem2 ==
  Ts : Inport  OutDataTypeStr=fixdt(0,32,32)
  Tx : Inport  Port=2  OutDataTypeStr=fixdt(0,32,30)
  Ty : Inport  Port=3  OutDataTypeStr=fixdt(0,32,30)
  Add : Sum  OutDataTypeStr=fixdt(0,32,32)
  Add1 : Sum  Inputs=-+  OutDataTypeStr=fixdt(1,32,4)
  Add2 : Sum  Inputs=+--  OutDataTypeStr=fixdt(0,32,32)
  Compare To Constant : simulink/Logic and Bit Operations/Compare To Constant  relop=>=  const=0  OutDataTypeStr=boolean
  Divide : Product  Inputs=*/  OutDataTypeStr=fixdt(0,32,20)
  Product : Product  OutDataTypeStr=fixdt(0,32,32)
  Switch : Switch  Criteria=u2 > Threshold  OutDataTypeStr=fixdt(0,32,33)
  Switch1 : Switch  Criteria=u2 > Threshold  OutDataTypeStr=fixdt(0,32,33)
  Tx_o : Outport
  Ty_o : Outport  Port=2
  wires:
  Compare To Constant/1 -> Switch/2, Switch1/2
  Add1/1 -> Switch1/3  "Ty'"
  Switch/1 -> Tx_o/1
  Switch1/1 -> Ty_o/1
  Add2/1 -> Compare To Constant/1
  Product/1 -> Add1/1, Switch/3  "Tx'"
  Divide/1 -> Product/1
  Tx/1 -> Add2/2, Add/1, Switch/1, Product/2
  Ts/1 -> Divide/1, Add2/1, Add1/2
  Add/1 -> Divide/2
  Ty/1 -> Add/2, Switch1/1, Add2/3

== system MtrCtrl_24V_2018/CurLpCtrl/Subsystem10/Subsystem/Cartesian to Polar ==
  In1 : Inport  LockScale=on
  In2 : Inport  Port=2  LockScale=on
  DTC_input_1 : DataTypeConversion  OutDataTypeStr=fixdt('double')  RndMeth=Nearest  LockScale=on
  DTC_input_2 : DataTypeConversion  OutDataTypeStr=fixdt('double')  RndMeth=Nearest  LockScale=on
  DTC_output_1 : DataTypeConversion  OutDataTypeStr=fixdt(0,32,32)
  DTC_output_2 : DataTypeConversion  OutDataTypeStr=fixdt(1,32,28)
  ReplicaOfSource : simulink_extras/Transformations/Cartesian to Polar
  Out1 : Outport  LockScale=on
  Out2 : Outport  Port=2  LockScale=on
  wires:
  DTC_output_2/1 -> Out2/1
  ReplicaOfSource/1 -> DTC_output_1/1
  DTC_output_1/1 -> Out1/1
  In1/1 -> DTC_input_1/1
  ReplicaOfSource/2 -> DTC_output_2/1
  In2/1 -> DTC_input_2/1
  DTC_input_2/1 -> ReplicaOfSource/2
  DTC_input_1/1 -> ReplicaOfSource/1

== system MtrCtrl_24V_2018/CurLpCtrl/Subsystem10/Subsystem/Polar to Cartesian ==
  In1 : Inport  LockScale=on
  In2 : Inport  Port=2  LockScale=on
  DTC_input_1 : DataTypeConversion  OutDataTypeStr=fixdt('double')  RndMeth=Nearest  LockScale=on
  DTC_input_2 : DataTypeConversion  OutDataTypeStr=fixdt('double')  RndMeth=Nearest  LockScale=on
  DTC_output_1 : DataTypeConversion  OutDataTypeStr=fixdt(1,32,31)
  DTC_output_2 : DataTypeConversion  OutDataTypeStr=fixdt(1,32,31)
  ReplicaOfSource : simulink_extras/Transformations/Polar to Cartesian
  Out1 : Outport  LockScale=on
  Out2 : Outport  Port=2  LockScale=on
  wires:
  In1/1 -> DTC_input_1/1
  ReplicaOfSource/2 -> DTC_output_2/1
  In2/1 -> DTC_input_2/1
  DTC_input_1/1 -> ReplicaOfSource/1
  ReplicaOfSource/1 -> DTC_output_1/1
  DTC_input_2/1 -> ReplicaOfSource/2
  DTC_output_1/1 -> Out1/1
  DTC_output_2/1 -> Out2/1

== system MtrCtrl_24V_2018/CurLpCtrl/Subsystem10/Subsystem/Subsystem1 ==
  vdq : Inport  OutDataTypeStr=fixdt(1,32,31)
  VphMax : Inport  Port=2  OutDataTypeStr=fixdt(0,32,32)
  Constant : Constant  Value=C_MATH_SqrtThreeOverThree_s32n31_Null
  Math Function : Math  Operator=square  OutDataTypeStr=fixdt(0,32,32)  SaturateOnIntegerOverflow=on
  Product : Product  OutDataTypeStr=Inherit: Inherit via back propagation
  Product1 : Product  Inputs=*/  OutDataTypeStr=fixdt(0,32,31)
  Scope : Scope  NumInputPorts=3
  Sqrt : Sqrt  OutDataTypeStr=fixdt(0,32,32)  SaturateOnIntegerOverflow=on
  Subsystem : Subsystem
  Sum of Elements : Sum  Inputs=+  OutDataTypeStr=fixdt(0,32,32)
  M : Outport  VectorParamsAs1DForOutWhenUnconnected=off
  wires:
  Sum of Elements/1 -> Sqrt/1
  Subsystem/1(OUT) -> Product1/2, Scope/3
  vdq/1 -> Math Function/1
  Math Function/1 -> Sum of Elements/1
  Product1/1 -> Scope/1, M/1
  Sqrt/1 -> Scope/2, Product1/1
  Product/1 -> Subsystem/1(IN)
  Constant/1 -> Product/2
  VphMax/1 -> Product/1

== system MtrCtrl_24V_2018/CurLpCtrl/Subsystem2/Z_alpha/If Action Subsystem ==
  In1 : Inport  OutDataTypeStr=fixdt(1,32,30)
  Action Port : ActionPort
  ZalphaOut : Outport
  wires:
  In1/1 -> ZalphaOut/1

== system MtrCtrl_24V_2018/CurLpCtrl/Subsystem2/Z_alpha/If Action Subsystem1 ==
  In1 : Inport  OutDataTypeStr=fixdt(1,32,30)
  Action Port : ActionPort
  ZalphaOut : Outport
  wires:
  In1/1 -> ZalphaOut/1

== system MtrCtrl_24V_2018/CurLpCtrl/Subsystem2/Z_alpha/If Action Subsystem2 ==
  In1 : Inport  OutDataTypeStr=fixdt(1,32,30)
  Action Port : ActionPort
  ZalphaOut : Outport
  wires:
  In1/1 -> ZalphaOut/1

== system MtrCtrl_24V_2018/CurLpCtrl/Subsystem2/Z_alpha1/If Action Subsystem ==
  In1 : Inport  OutDataTypeStr=fixdt(1,32,30)
  Action Port : ActionPort
  ZalphaOut : Outport
  wires:
  In1/1 -> ZalphaOut/1

== system MtrCtrl_24V_2018/CurLpCtrl/Subsystem2/Z_alpha1/If Action Subsystem1 ==
  In1 : Inport  OutDataTypeStr=fixdt(1,32,30)
  Action Port : ActionPort
  ZalphaOut : Outport
  wires:
  In1/1 -> ZalphaOut/1

== system MtrCtrl_24V_2018/CurLpCtrl/Subsystem2/Z_alpha1/If Action Subsystem2 ==
  In1 : Inport  OutDataTypeStr=fixdt(1,32,30)
  Action Port : ActionPort
  ZalphaOut : Outport
  wires:
  In1/1 -> ZalphaOut/1

== system MtrCtrl_24V_2018/CurLpCtrl/Subsystem8/F9/F2 ==
  Id_k : Inport
  Iq_k : Inport  Port=2
  we : Inport  Port=3
  Ud_k : Inport  Port=4
  Uq_k : Inport  Port=5
  Add{2..5} (4 alike) : Sum
  Constant1 : Constant  Value=1-TsCtrl*Rs/Ls
  Constant2 : Constant  Value=TsCtrl/Ls
  Constant3 : Constant  Value=1-TsCtrl*Rs/Ls
  Constant4 : Constant  Value=TsCtrl/Ls
  Gain6 : Gain  Gain=TsCtrl
  Gain7 : Gain  Gain=-1
  Product{5,9..13} (6 alike) : Product
  Id_k_1 : Outport
  Iq_k_1 : Outport  Port=2
  wires:
  Gain6/1 -> Gain7/1, Product9/2
  Product11/1 -> Add3/2
  Add3/1 -> Add5/1
  we/1 -> Gain6/1
  Add2/1 -> Add4/1
  Product5/1 -> Add2/1
  Constant2/1 -> Product13/1
  Product12/1 -> Add4/2
  Gain7/1 -> Product10/1
  Product9/1 -> Add2/2
  Product13/1 -> Add5/2
  Iq_k/1 -> Product9/1, Product11/2
  Constant4/1 -> Product12/1
  Product10/1 -> Add3/1
  Constant3/1 -> Product5/2
  Constant1/1 -> Product11/1
  Ud_k/1 -> Product12/2
  Uq_k/1 -> Product13/2
  Id_k/1 -> Product10/2, Product5/1
  Add4/1 -> Id_k_1/1  "Id_k_1"
  Add5/1 -> Iq_k_1/1  "Iq_k_1"

== system MtrCtrl_24V_2018/CurLpCtrl/Subsystem8/F9/F8 ==
  Id_k1 : Inport
  Iq_k1 : Inport  Port=2
  we : Inport  Port=3
  Ud_k1 : Inport  Port=4
  Uq_k1 : Inport  Port=5
  Add1 : Sum
  Add6 : Sum
  Add7 : Sum
  Add8 : Sum  Inputs=++-
  Constant : Constant  Value=Flux/Ls
  Constant5 : Constant  Value=1-TsCtrl*Rs/Ls
  Constant6 : Constant  Value=TsCtrl/Ls
  Constant7 : Constant  Value=1-TsCtrl*Rs/Ls
  Constant8 : Constant  Value=TsCtrl/Ls
  Gain1 : Gain  Gain=TsCtrl
  Gain2 : Gain  Gain=-1
  Product{1..7} (7 alike) : Product
  Id_k : Outport
  Iq_k : Outport  Port=2
  wires:
  Id_k1/1 -> Product1/2, Product6/1
  Product2/1 -> Add6/2
  Add1/1 -> Add7/1
  Constant7/1 -> Product6/2
  Product6/1 -> Add1/1
  Ud_k1/1 -> Product3/2
  Iq_k1/1 -> Product2/2, Product7/1
  Constant5/1 -> Product2/1
  Product1/1 -> Add6/1
  Product3/1 -> Add7/2
  Gain2/1 -> Product5/1, Product1/1
  Constant8/1 -> Product3/1
  Constant6/1 -> Product4/1
  Product4/1 -> Add8/2
  Product7/1 -> Add1/2
  Add6/1 -> Add8/1
  Gain1/1 -> Gain2/1, Product7/2
  we/1 -> Gain1/1
  Uq_k1/1 -> Product4/2
  Add7/1 -> Id_k/1  "Id_k"
  Add8/1 -> Iq_k/1  "Iq_k"
  Product5/1 -> Add8/3
  Constant/1 -> Product5/2

== system MtrCtrl_24V_2018/CurLpCtrl/Subsystem10/Subsystem/Subsystem1/Subsystem ==
  IN : Inport  OutDataTypeStr=fixdt(0,32,32)
  Constant2 : Constant  Value=0.1  OutDataTypeStr=fixdt(0,32,32)  SampleTime=-1
  Switch : Switch  Criteria=u2 > Threshold  Threshold=0.1  OutDataTypeStr=fixdt(0,32,32)
  OUT : Outport  VectorParamsAs1DForOutWhenUnconnected=off
  wires:
  IN/1 -> Switch/2, Switch/1
  Constant2/1 -> Switch/3
  Switch/1 -> OUT/1

== stateflow chart MtrCtrl_24V_2018/CurLpCtrl/SVPWM/Overmodulation/Chart ==
  (default) -> (junction 2)
  (junction 2) -> (junction 4) [order 1] : [Tx+Ty >= Ts*TwoTimeSqrtThreeOverThree]
  (junction 4) -> (junction 6) [order 1] : [Tx>Ty]
  (junction 2) -> (junction 29) [order 2] : {
      | Tx_o = Tx;
      | Ty_o = Ty;
      | }
  (junction 4) -> (junction 1) [order 2]
  (junction 6) -> (junction 9) : {
      | Tx_o = Ts;
      | Ty_o = 0;
      | }
  (junction 1) -> (junction 12) [order 1] : [Ty > Tx]
  (junction 1) -> (junction 16) [order 2]
  (junction 12) -> (junction 14) : {
      | Tx_o = 0;
      | Ty_o = Ts;
      | }
  (junction 16) -> (junction 18) [order 1] : [Ty > Ts && Ts > Tx]
  (junction 16) -> (junction 25) [order 2] : {
      | m = Ts/(Tx+Ty);
      | Tx_o = Tx * m;
      | Ty_o = Ty * m;
      | }
  (junction 18) -> (junction 20) : {
      | Tx_o = 0;
      | Ty_o = Ts;
      | }
  (junction 25) -> (junction 29)
  (junction 20) -> (junction 25)
  (junction 14) -> (junction 20)
  (junction 9) -> (junction 14)
  data: Tx_o output fixdt(0,32,30); Ts input; Ty input; Ty_o output fixdt(0,32,30); Tx input; m local fixdt(1,32,4) size=1 =1; TwoTimeSqrtThreeOverThree local fixdt(0,32,30) size=1 =1.15470053814351558685302734375
